simulink library "magnetometer_lib"  (R2018b)
settings: Solver=VariableStepAuto  StartTime=0.0  StopTime=10.0  RelTol=1e-3
undefined symbols (not defined in the file): simParams
libraries: simulink x3, dspmathops x2, aerolibutil x1
settings Model: Creator=colem  LastModifiedBy=taylorreynolds

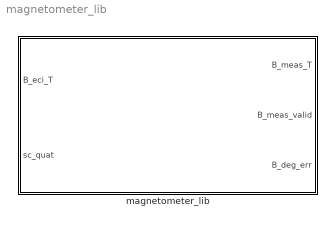
== system magnetometer_lib ==
  magnetometer_lib : Subsystem  mask{id_s=1}
      mask prompts: id_s "Choose the sensor ID"
      mask TypeOptions id_s: 1 | 2 | 3
      mask DialogControl DescTextVar Prompt: SOCi magnetometer model. The spacecraft has three Honeywell HMC5993 magnetometers.

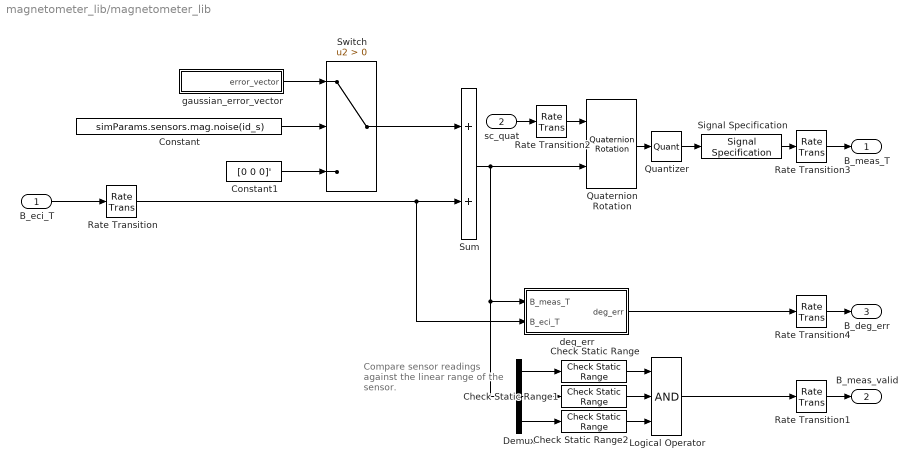
== system magnetometer_lib/magnetometer_lib ==
  note: Compare sensor readings
      | against the linear range
      | of the sensor.
  B_eci_T : Inport
  sc_quat : Inport  Port=2
  Check Static Range : simulink/Model Verification/Check  Static Range  Description=simParams.sensors.mag.B_min(id_s) <= u <= simParams.sensors.mag.B_max(id_s)  max=simParams.sensors.mag.B_max(id_s)  max_included=on  min=simParams.sensors.mag.B_min(id_s)  min_included=on  enabled=on  stopWhenAssertionFail=off  export=on  icon=text
      settings: SourceProductName=Simulink  SourceProductBaseCode=SL
  Check Static Range1 : simulink/Model Verification/Check  Static Range  Description=simParams.sensors.mag.B_min(id_s) <= u <= simParams.sensors.mag.B_max(id_s)  max=simParams.sensors.mag.B_max(id_s)  max_included=on  min=simParams.sensors.mag.B_min(id_s)  min_included=on  enabled=on  stopWhenAssertionFail=off  export=on  icon=text
      settings: SourceProductName=Simulink  SourceProductBaseCode=SL
  Check Static Range2 : simulink/Model Verification/Check  Static Range  Description=simParams.sensors.mag.B_min(id_s) <= u <= simParams.sensors.mag.B_max(id_s)  max=simParams.sensors.mag.B_max(id_s)  max_included=on  min=simParams.sensors.mag.B_min(id_s)  min_included=on  enabled=on  stopWhenAssertionFail=off  export=on  icon=text
      settings: SourceProductName=Simulink  SourceProductBaseCode=SL
  Constant : Constant  Value=simParams.sensors.mag.noise(id_s)  SampleTime=simParams.sensors.mag.sample_time_s
  Constant1 : Constant  Value=[0 0 0]'
  Demux : Demux  Outputs=3
  Logical Operator : Logic  Inputs=3  AllPortsSameDT=off  OutDataTypeStr=boolean
  Quantizer : Quantizer  QuantizationInterval=simParams.sensors.mag.resolution(id_s)
  Quaternion Rotation : aerolibutil/Quaternion Rotation
  Rate Transition : RateTransition  InitialCondition=simParams.sensors.mag.ic.B_eci_T  OutPortSampleTime=simParams.sensors.mag.sample_time_s
  Rate Transition1 : RateTransition
  Rate Transition2 : RateTransition  InitialCondition=simParams.initialConditions.q_eci2body  OutPortSampleTime=simParams.sensors.mag.sample_time_s
  Rate Transition3 : RateTransition  InitialCondition=simParams.sensors.mag.ic.B_eci_T
  Rate Transition4 : RateTransition
  Signal Specification : SignalSpecification  Dimensions=3
  Sum : Sum
  Switch : Switch  Criteria=u2 > Threshold
  deg_err : Subsystem
  gaussian_error_vector : Subsystem
  B_meas_T : Outport
  B_meas_valid : Outport  Port=2
  B_deg_err : Outport  Port=3
  wires:
  sc_quat/1 -> Rate Transition2/1
  Switch/1 -> Sum/1
  Constant/1 -> Switch/2
  Sum/1 -> Quaternion Rotation/2, deg_err/1(B_meas_T), Demux/1
  Constant1/1 -> Switch/3
  gaussian_error_vector/1(error_vector) -> Switch/1
  B_eci_T/1 -> Rate Transition/1
  deg_err/1(deg_err) -> Rate Transition4/1
  Rate Transition/1 -> deg_err/2(B_eci_T), Sum/2
  Rate Transition1/1 -> B_meas_valid/1
  Rate Transition2/1 -> Quaternion Rotation/1
  Rate Transition3/1 -> B_meas_T/1
  Quaternion Rotation/1 -> Quantizer/1
  Rate Transition4/1 -> B_deg_err/1
  Quantizer/1 -> Signal Specification/1
  Demux/1 -> Check Static Range/1
  Demux/2 -> Check Static Range1/1
  Demux/3 -> Check Static Range2/1
  Check Static Range/1 -> Logical Operator/1
  Check Static Range1/1 -> Logical Operator/2
  Check Static Range2/1 -> Logical Operator/3
  Logical Operator/1 -> Rate Transition1/1
  Signal Specification/1 -> Rate Transition3/1

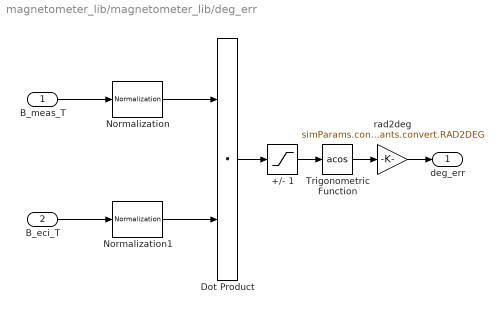
== system magnetometer_lib/magnetometer_lib/deg_err ==
  B_meas_T : Inport
  B_eci_T : Inport  Port=2
  +/- 1 : Saturate  UpperLimit=1  LowerLimit=-1
  Dot Product : DotProduct  InputSameDT=on  OutDataTypeStr=Inherit: Inherit via internal rule
  Normalization : dspmathops/Normalization  NormType=2-norm  Bias=1e-10  NormOver=Each column  Dimension=1  roundingMode=Floor  overflowMode=off  accumDataTypeStr=Inherit: Same as product output  accumLastDataTypeStr=Inherit: Same as product output  outputDataTypeStr=Inherit: Same as product output  outputMin=[]  outputMax=[]  outputLastDataTypeStr=Inherit: Same as product output
      settings: SourceProductName=DSP System Toolbox
  Normalization1 : dspmathops/Normalization  NormType=2-norm  Bias=1e-10  NormOver=Each column  Dimension=1  roundingMode=Floor  overflowMode=off  accumDataTypeStr=Inherit: Same as product output  accumLastDataTypeStr=Inherit: Same as product output  outputDataTypeStr=Inherit: Same as product output  outputMin=[]  outputMax=[]  outputLastDataTypeStr=Inherit: Same as product output
      settings: SourceProductName=DSP System Toolbox
  Trigonometric Function : Trigonometry  Operator=acos
  rad2deg : Gain  Gain=simParams.constants.convert.RAD2DEG
  deg_err : Outport
  wires:
  B_meas_T/1 -> Normalization/1
  Normalization/1 -> Dot Product/1
  B_eci_T/1 -> Normalization1/1
  Normalization1/1 -> Dot Product/2
  Dot Product/1 -> +/- 1/1
  Trigonometric Function/1 -> rad2deg/1
  +/- 1/1 -> Trigonometric Function/1
  rad2deg/1 -> deg_err/1

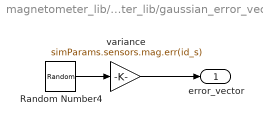
== system magnetometer_lib/magnetometer_lib/gaussian_error_vector ==
  Random Number4 : RandomNumber  Mean=[0;0;0]  Variance=[1;1;1]  Seed=simParams.sensors.mag.seed(:,id_s)  SampleTime=simParams.sensors.mag.sample_time_s
  variance : Gain  Gain=simParams.sensors.mag.err(id_s)
  error_vector : Outport
  wires:
  Random Number4/1 -> variance/1
  variance/1 -> error_vector/1
